simulink model "mapp_4_fir_4_str"  (R2018b)
settings: Solver=ode45  StartTime=0.0  StopTime=200  RelTol=1e-3  EnableMultiTasking=on
undefined symbols (not defined in the file or in its folder): CMD_ci_Re_0, CMD_ci_Re_21, CMD_ci_str_0, CMD_ci_str_1, CMD_ci_str_10, CMD_ci_str_11, CMD_ci_str_12, CMD_ci_str_13, CMD_ci_str_14, CMD_ci_str_15, CMD_ci_str_16, CMD_ci_str_17, CMD_ci_str_18, CMD_ci_str_19, CMD_ci_str_2, CMD_ci_str_20, CMD_ci_str_21, CMD_ci_str_3, CMD_ci_str_4, CMD_ci_str_5, CMD_ci_str_6, CMD_ci_str_7, CMD_ci_str_8, CMD_ci_str_9, CMD_decr_0, CMD_deka_down, CMD_deka_up, CMD_fb, CMD_FB_mult, CMD_Firprg_0, CMD_Firprg_1, CMD_gain, CMD_ind_mult, CMD_ind_mult_1, CMD_ind_mult_2, CMD_ind_mult_3, CMD_ind_mult_4, CMD_ind_stuk, CMD_ind_vol, CMD_ind_vol_1, CMD_ind_vol_2, CMD_ind_vol_3, CMD_ind_vol_4, CMD_init_dac, CMD_init_sw, CMD_molot_string, CMD_nl, CMD_nl_sl, CMD_omega_0, CMD_out_vol, CMD_param_0, CMD_param_5, CMD_pedal, CMD_reset, CMD_rst, CMD_shape_0, CMD_step_down, CMD_step_up, CMD_str_svertk, ind_mult_0 ... (+10)
libraries: xbsIndex_r4 x3300
(part 4 of 16)

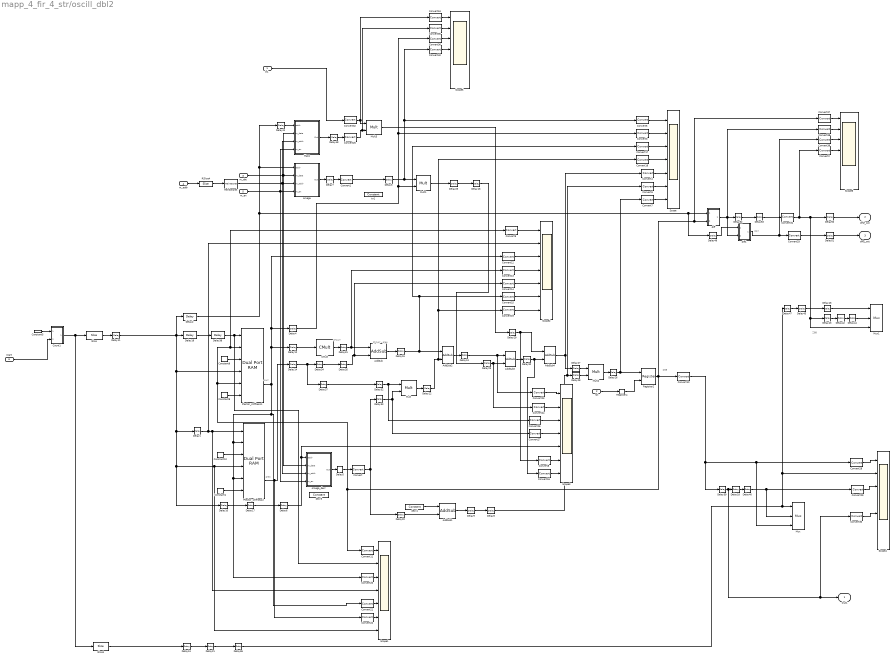
== system mapp_4_fir_4_str/oscill_dbl2 ==
  note: 2*curr - prev
  note: prev
  note: curr
  note: 2*curr
  note: Z59
  note: Z17
  note: Z88
  In1 : Inport
  rst : Inport  Port=2
  m_dat : Inport  Port=3
  m_addr : Inport  Port=4
  m_en : Inport  Port=5
  start : Inport  Port=6
  AddSub : xbsIndex_r4/AddSub  mode=Subtraction  use_carryin=off  use_carryout=off  en=off  latency=11  precision=Full  arith_type=Unsigned  n_bits=16  bin_pt=14  quantization=Truncate  overflow=Wrap  use_behavioral_HDL=off  hw_selection=DSP48  pipelined=on  dbl_ovrd=off  block_type=addsub
  AddSub1 : xbsIndex_r4/AddSub  mode=Subtraction  use_carryin=off  use_carryout=off  en=off  latency=11  precision=Full  arith_type=Unsigned  n_bits=25  bin_pt=0  quantization=Truncate  overflow=Wrap  use_behavioral_HDL=off  hw_selection=Fabric  pipelined=off  dbl_ovrd=off  block_type=addsub
  AddSub2 : xbsIndex_r4/AddSub  mode=Addition  use_carryin=off  use_carryout=off  en=off  latency=11  precision=Full  arith_type=Unsigned  n_bits=16  bin_pt=14  quantization=Truncate  overflow=Wrap  use_behavioral_HDL=off  hw_selection=Fabric  pipelined=off  dbl_ovrd=off  block_type=addsub
  AddSub3 : xbsIndex_r4/AddSub  mode=Subtraction  use_carryin=off  use_carryout=off  en=off  latency=11  precision=Full  arith_type=Unsigned  n_bits=16  bin_pt=14  quantization=Truncate  overflow=Wrap  use_behavioral_HDL=off  hw_selection=Fabric  pipelined=off  dbl_ovrd=off  block_type=addsub
  AddSub4 : xbsIndex_r4/AddSub  mode=Addition  use_carryin=off  use_carryout=off  en=off  latency=11  precision=Full  arith_type=Unsigned  n_bits=16  bin_pt=14  quantization=Truncate  overflow=Wrap  use_behavioral_HDL=off  hw_selection=Fabric  pipelined=off  dbl_ovrd=off  block_type=addsub
  CMult : xbsIndex_r4/CMult  const=2  gui_display_data_type=Floating-point  const_n_bits=16  const_bin_pt=14  float_type=Double  exp_bits=8  fraction_bits=24  en=off  latency=8  precision=Full  arith_type="Signed  (2's comp)"  n_bits=16  bin_pt=14  quantization=Truncate  overflow=Wrap  use_behavioral_HDL=off  mem_type=Distributed RAM  pipeline=on  dbl_ovrd=off  block_type=cmult
  Constant1 : xbsIndex_r4/Constant  const=0  gui_display_data_type=Boolean  arith_type=Boolean  n_bits=18  bin_pt=0  preci_type=Single  exp_width=8  frac_width=24  explicit_period=on  period=1  equ=P=C  opselect=C  inp2=PCIN>>17  opr=+  inp1=P  carry=CIN  dbl_ovrd=off  block_type=constant
      settings: block_version=VER_STRING_GOES_HERE
  Constant10 : xbsIndex_r4/Constant  const=1  gui_display_data_type=Boolean  arith_type=Boolean  n_bits=18  bin_pt=0  preci_type=Single  exp_width=8  frac_width=24  explicit_period=on  period=1  equ=P=C  opselect=C  inp2=PCIN>>17  opr=+  inp1=P  carry=CIN  dbl_ovrd=off  block_type=constant
      settings: block_version=VER_STRING_GOES_HERE
  Constant5 : xbsIndex_r4/Constant  const=169  gui_display_data_type=Fixed-point  arith_type=Unsigned  n_bits=12  bin_pt=0  preci_type=Single  exp_width=8  frac_width=24  explicit_period=off  period=1  equ=P=C  opselect=C  inp2=PCIN>>17  opr=+  inp1=P  carry=CIN  dbl_ovrd=off  block_type=constant
      settings: block_version=VER_STRING_GOES_HERE
  Constant8 : xbsIndex_r4/Constant  const=0  gui_display_data_type=Boolean  arith_type=Boolean  n_bits=18  bin_pt=0  preci_type=Single  exp_width=8  frac_width=24  explicit_period=on  period=1  equ=P=C  opselect=C  inp2=PCIN>>17  opr=+  inp1=P  carry=CIN  dbl_ovrd=off  block_type=constant
      settings: block_version=VER_STRING_GOES_HERE
  Constant9 : xbsIndex_r4/Constant  const=1  gui_display_data_type=Boolean  arith_type=Boolean  n_bits=18  bin_pt=0  preci_type=Single  exp_width=8  frac_width=24  explicit_period=on  period=1  equ=P=C  opselect=C  inp2=PCIN>>17  opr=+  inp1=P  carry=CIN  dbl_ovrd=off  block_type=constant
      settings: block_version=VER_STRING_GOES_HERE
  Convert{,1,25,32} (4 alike) : xbsIndex_r4/Convert  gui_display_data_type=Floating-point  arith_type=Floating-point  n_bits=16  bin_pt=14  float_type=Double  exp_bits=8  fraction_bits=24  quantization=Truncate  overflow=Wrap  en=off  latency=12  pipeline=off  dbl_ovrd=off  block_type=convert
  Convert10 : xbsIndex_r4/Convert  gui_display_data_type=Floating-point  arith_type=Floating-point  n_bits=16  bin_pt=14  float_type=Single  exp_bits=8  fraction_bits=24  quantization=Truncate  overflow=Wrap  en=off  latency=12  pipeline=off  dbl_ovrd=off  block_type=convert
  Convert{3..9,11..24,26..27,34..40} (30 alike) : xbsIndex_r4/Convert  gui_display_data_type=Floating-point  arith_type=Floating-point  n_bits=16  bin_pt=14  float_type=Double  exp_bits=8  fraction_bits=24  quantization=Truncate  overflow=Wrap  en=off  latency=0  pipeline=off  dbl_ovrd=off  block_type=convert
  Convert{2,28..30} (4 alike) : xbsIndex_r4/Convert  gui_display_data_type=Floating-point  arith_type=Floating-point  n_bits=16  bin_pt=14  float_type=Single  exp_bits=8  fraction_bits=24  quantization=Truncate  overflow=Wrap  en=off  latency=0  pipeline=off  dbl_ovrd=off  block_type=convert
  Convert31 : xbsIndex_r4/Convert  gui_display_data_type=Floating-point  arith_type=Floating-point  n_bits=16  bin_pt=14  float_type=Single  exp_bits=8  fraction_bits=24  quantization=Truncate  overflow=Wrap  en=off  latency=12  pipeline=off  dbl_ovrd=off  block_type=convert
  Convert33 : xbsIndex_r4/Convert  gui_display_data_type=Floating-point  arith_type=Floating-point  n_bits=16  bin_pt=14  float_type=Single  exp_bits=8  fraction_bits=24  quantization=Truncate  overflow=Wrap  en=off  latency=12  pipeline=off  dbl_ovrd=off  block_type=convert
  Count1 : Subsystem
  Delay{1,3,16,33} (4 alike) : xbsIndex_r4/Delay  rst=off  infoeditControl=Selection of Reset will increase slice count due to use of real FFs and instead of SRLs  en=off  latency=2  reg_retiming=on  dbl_ovrd=off  block_type=delay
      settings: xl_area=[16 32 0 0 0 0 0]  block_version=VER_STRING_GOES_HERE
  Delay{2,5..7,9..10,12..15,22..32,35..36,38..40,43..44,46..48,50..51,53} (34 alike) : xbsIndex_r4/Delay  rst=off  infoeditControl=Selection of Reset will increase slice count due to use of real FFs and instead of SRLs  en=off  latency=1  reg_retiming=on  dbl_ovrd=off  block_type=delay
      Delay10 settings: xl_area=[16 32 0 0 0 0 0]  block_version=VER_STRING_GOES_HERE
      Delay12 settings: xl_area=[16 32 0 0 0 0 0]  block_version=VER_STRING_GOES_HERE
      Delay13 settings: xl_area=[16 32 0 0 0 0 0]  block_version=VER_STRING_GOES_HERE
      Delay14 settings: xl_area=[16 32 0 0 0 0 0]  block_version=VER_STRING_GOES_HERE
      Delay15 settings: xl_area=[16 32 0 0 0 0 0]  block_version=VER_STRING_GOES_HERE
      Delay2 settings: xl_area=[1 1 0 0 0 0 0]  block_version=8.2-EVAL
      Delay22 settings: xl_area=[16 32 0 0 0 0 0]  block_version=VER_STRING_GOES_HERE
      Delay23 settings: xl_area=[16 32 0 0 0 0 0]  block_version=VER_STRING_GOES_HERE
      Delay24 settings: xl_area=[16 32 0 0 0 0 0]  block_version=VER_STRING_GOES_HERE
      Delay25 settings: xl_area=[16 32 0 0 0 0 0]  block_version=VER_STRING_GOES_HERE
      Delay26 settings: xl_area=[16 32 0 0 0 0 0]  block_version=VER_STRING_GOES_HERE
      Delay27 settings: xl_area=[16 32 0 0 0 0 0]  block_version=VER_STRING_GOES_HERE
      Delay28 settings: xl_area=[16 32 0 0 0 0 0]  block_version=VER_STRING_GOES_HERE
      Delay29 settings: xl_area=[16 32 0 0 0 0 0]  block_version=VER_STRING_GOES_HERE
      Delay30 settings: xl_area=[16 32 0 0 0 0 0]  block_version=VER_STRING_GOES_HERE
      Delay31 settings: xl_area=[16 32 0 0 0 0 0]  block_version=VER_STRING_GOES_HERE
      Delay32 settings: xl_area=[16 32 0 0 0 0 0]  block_version=VER_STRING_GOES_HERE
      Delay35 settings: xl_area=[16 32 0 0 0 0 0]  block_version=VER_STRING_GOES_HERE
      Delay36 settings: xl_area=[16 32 0 0 0 0 0]  block_version=VER_STRING_GOES_HERE
      Delay38 settings: xl_area=[1 1 0 0 0 0 0]  block_version=8.2-EVAL
      Delay39 settings: xl_area=[16 32 0 0 0 0 0]  block_version=VER_STRING_GOES_HERE
      Delay40 settings: xl_area=[16 32 0 0 0 0 0]  block_version=VER_STRING_GOES_HERE
      Delay43 settings: xl_area=[16 32 0 0 0 0 0]  block_version=VER_STRING_GOES_HERE
      Delay44 settings: xl_area=[16 32 0 0 0 0 0]  block_version=VER_STRING_GOES_HERE
      Delay46 settings: xl_area=[16 32 0 0 0 0 0]  block_version=VER_STRING_GOES_HERE
      Delay47 settings: xl_area=[16 32 0 0 0 0 0]  block_version=VER_STRING_GOES_HERE
      Delay48 settings: xl_area=[16 32 0 0 0 0 0]  block_version=VER_STRING_GOES_HERE
      Delay5 settings: xl_area=[16 32 0 0 0 0 0]  block_version=VER_STRING_GOES_HERE
      Delay50 settings: xl_area=[16 32 0 0 0 0 0]  block_version=VER_STRING_GOES_HERE
      Delay51 settings: xl_area=[16 32 0 0 0 0 0]  block_version=VER_STRING_GOES_HERE
      Delay53 settings: xl_area=[16 32 0 0 0 0 0]  block_version=VER_STRING_GOES_HERE
      Delay6 settings: xl_area=[16 32 0 0 0 0 0]  block_version=VER_STRING_GOES_HERE
      Delay7 settings: xl_area=[16 32 0 0 0 0 0]  block_version=VER_STRING_GOES_HERE
      Delay9 settings: xl_area=[16 32 0 0 0 0 0]  block_version=VER_STRING_GOES_HERE
  Delay11 : xbsIndex_r4/Delay  rst=off  infoeditControl=Selection of Reset will increase slice count due to use of real FFs and instead of SRLs  en=off  latency=16  reg_retiming=on  dbl_ovrd=off  block_type=delay
      settings: xl_area=[16 32 0 0 0 0 0]  block_version=VER_STRING_GOES_HERE
  Delay17 : xbsIndex_r4/Delay  rst=off  infoeditControl=Selection of Reset will increase slice count due to use of real FFs and instead of SRLs  en=off  latency=246  reg_retiming=on  dbl_ovrd=off  block_type=delay
      settings: xl_area=[16 32 0 0 0 0 0]  block_version=VER_STRING_GOES_HERE
  Delay18 : xbsIndex_r4/Delay  rst=off  infoeditControl=Selection of Reset will increase slice count due to use of real FFs and instead of SRLs  en=off  latency=254  reg_retiming=on  dbl_ovrd=off  block_type=delay
      settings: xl_area=[16 32 0 0 0 0 0]  block_version=VER_STRING_GOES_HERE
  Delay19 : xbsIndex_r4/Delay  rst=off  infoeditControl=Selection of Reset will increase slice count due to use of real FFs and instead of SRLs  en=off  latency=77  reg_retiming=on  dbl_ovrd=off  block_type=delay
      settings: xl_area=[1 1 0 0 0 0 0]  block_version=8.2-EVAL
  Delay20 : xbsIndex_r4/Delay  rst=off  infoeditControl=Selection of Reset will increase slice count due to use of real FFs and instead of SRLs  en=off  latency=12  reg_retiming=on  dbl_ovrd=off  block_type=delay
      settings: xl_area=[16 32 0 0 0 0 0]  block_version=VER_STRING_GOES_HERE
  Delay21 : xbsIndex_r4/Delay  rst=off  infoeditControl=Selection of Reset will increase slice count due to use of real FFs and instead of SRLs  en=off  latency=41 + 64  reg_retiming=on  dbl_ovrd=off  block_type=delay
      settings: xl_area=[16 32 0 0 0 0 0]  block_version=VER_STRING_GOES_HERE
  Delay34 : xbsIndex_r4/Delay  rst=off  infoeditControl=Selection of Reset will increase slice count due to use of real FFs and instead of SRLs  en=off  latency=8  reg_retiming=on  dbl_ovrd=off  block_type=delay
      settings: xl_area=[16 32 0 0 0 0 0]  block_version=VER_STRING_GOES_HERE
  Delay37 : xbsIndex_r4/Delay  rst=off  infoeditControl=Selection of Reset will increase slice count due to use of real FFs and instead of SRLs  en=off  latency=3  reg_retiming=on  dbl_ovrd=off  block_type=delay
      settings: xl_area=[16 32 0 0 0 0 0]  block_version=VER_STRING_GOES_HERE
  Delay4 : xbsIndex_r4/Delay  rst=off  infoeditControl=Selection of Reset will increase slice count due to use of real FFs and instead of SRLs  en=off  latency=14  reg_retiming=on  dbl_ovrd=off  block_type=delay
      settings: xl_area=[16 32 0 0 0 0 0]  block_version=VER_STRING_GOES_HERE
  Delay41 : xbsIndex_r4/Delay  rst=off  infoeditControl=Selection of Reset will increase slice count due to use of real FFs and instead of SRLs  en=off  latency=17  reg_retiming=on  dbl_ovrd=off  block_type=delay
      settings: xl_area=[16 32 0 0 0 0 0]  block_version=VER_STRING_GOES_HERE
  Delay42 : xbsIndex_r4/Delay  rst=off  infoeditControl=Selection of Reset will increase slice count due to use of real FFs and instead of SRLs  en=off  latency=126  reg_retiming=on  dbl_ovrd=off  block_type=delay
      settings: xl_area=[16 32 0 0 0 0 0]  block_version=VER_STRING_GOES_HERE
  Delay45 : xbsIndex_r4/Delay  rst=off  infoeditControl=Selection of Reset will increase slice count due to use of real FFs and instead of SRLs  en=off  latency=15  reg_retiming=on  dbl_ovrd=off  block_type=delay
      settings: xl_area=[16 32 0 0 0 0 0]  block_version=VER_STRING_GOES_HERE
  Delay49 : xbsIndex_r4/Delay  rst=off  infoeditControl=Selection of Reset will increase slice count due to use of real FFs and instead of SRLs  en=off  latency=17  reg_retiming=on  dbl_ovrd=off  block_type=delay
      settings: xl_area=[16 32 0 0 0 0 0]  block_version=VER_STRING_GOES_HERE
  Delay52 : xbsIndex_r4/Delay  rst=off  infoeditControl=Selection of Reset will increase slice count due to use of real FFs and instead of SRLs  en=off  latency=16  reg_retiming=on  dbl_ovrd=off  block_type=delay
      settings: xl_area=[16 32 0 0 0 0 0]  block_version=VER_STRING_GOES_HERE
  Delay8 : xbsIndex_r4/Delay  rst=off  infoeditControl=Selection of Reset will increase slice count due to use of real FFs and instead of SRLs  en=off  latency=30  reg_retiming=on  dbl_ovrd=off  block_type=delay
      settings: xl_area=[16 32 0 0 0 0 0]  block_version=VER_STRING_GOES_HERE
  Mass : Subsystem
  Mult : xbsIndex_r4/Mult  precision=Full  arith_type="Signed  (2's comp)"  n_bits=48  bin_pt=48  quantization=Truncate  overflow=Wrap  en=off  latency=16  use_behavioral_HDL=off  opt=Speed  use_embedded=on  optimum_pipeline=on  pipeline=on  dbl_ovrd=off  use_rpm=on  placement_style=Triangular  block_type=mult
      settings: block_version=9.1.01-EVAL
  Mult1 : xbsIndex_r4/Mult  precision=Full  arith_type="Signed  (2's comp)"  n_bits=48  bin_pt=48  quantization=Truncate  overflow=Wrap  en=off  latency=16  use_behavioral_HDL=on  opt=Speed  use_embedded=on  optimum_pipeline=on  pipeline=on  dbl_ovrd=off  use_rpm=on  placement_style=Triangular  block_type=mult
      settings: block_version=9.1.01-EVAL
  Mult2 : xbsIndex_r4/Mult  precision=Full  arith_type="Signed  (2's comp)"  n_bits=48  bin_pt=48  quantization=Truncate  overflow=Wrap  en=off  latency=16  use_behavioral_HDL=on  opt=Speed  use_embedded=on  optimum_pipeline=on  pipeline=on  dbl_ovrd=off  use_rpm=on  placement_style=Triangular  block_type=mult
      settings: block_version=9.1.01-EVAL
  Mult3 : xbsIndex_r4/Mult  precision=Full  arith_type="Signed  (2's comp)"  n_bits=48  bin_pt=48  quantization=Truncate  overflow=Wrap  en=off  latency=16  use_behavioral_HDL=on  opt=Speed  use_embedded=on  optimum_pipeline=on  pipeline=on  dbl_ovrd=off  use_rpm=on  placement_style=Triangular  block_type=mult
      settings: block_version=9.1.01-EVAL
  Mux : xbsIndex_r4/Mux  inputs=2  en=off  latency=0  precision=Full  arith_type=Unsigned  n_bits=16  bin_pt=14  quantization=Truncate  overflow=Wrap  dbl_ovrd=off  block_type=mux
  Mux1 : xbsIndex_r4/Mux  inputs=2  en=off  latency=0  precision=Full  arith_type=Unsigned  n_bits=16  bin_pt=14  quantization=Truncate  overflow=Wrap  dbl_ovrd=off  block_type=mux
  Plector_stiffness1 : xbsIndex_r4/Dual Port RAM  depth=256  initVector=zeros  distributed_mem=Block RAM  init_a=0  init_b=0  rst_a=off  rst_b=off  en_a=off  en_b=off  latency=2  write_mode_A=Read Before Write  write_mode_B=Read Before Write  optimize=Area  dbl_ovrd=off  block_type=dpram
      settings: block_version=10.1.1
  Plector_stiffness2 : xbsIndex_r4/Dual Port RAM  depth=256  initVector=zeros  distributed_mem=Block RAM  init_a=0  init_b=0  rst_a=off  rst_b=off  en_a=off  en_b=off  latency=2  write_mode_A=Read Before Write  write_mode_B=Read Before Write  optimize=Area  dbl_ovrd=off  block_type=dpram
      settings: block_version=10.1.1
  RSlice4 : xbsIndex_r4/Slice  nbits=8  boolean_output=off  mode=Lower Bit Location + Width  bit1=0  base1=MSB of Input  bit0=0  base0=LSB of Input  dbl_ovrd=off  block_type=slice
      settings: block_version=VER_STRING_GOES_HERE
  Register2 : xbsIndex_r4/Register  init=0  rst=on  en=off  dbl_ovrd=off  block_type=register
  Register4 : xbsIndex_r4/Register  init=0  rst=off  en=off  dbl_ovrd=off  block_type=register
  Reinterpret : xbsIndex_r4/Reinterpret  force_arith_type=off  arith_type=Unsigned  force_bin_pt=off  bin_pt=0  block_type=reinterpret
  Scope{,1..6} (7 alike) : Scope  NumInputPorts=7
  Slice : xbsIndex_r4/Slice  nbits=8  boolean_output=off  mode=Lower Bit Location + Width  bit1=0  base1=MSB of Input  bit0=0  base0=LSB of Input  dbl_ovrd=off  block_type=slice
  Slice1 : xbsIndex_r4/Slice  nbits=1  boolean_output=off  mode=Lower Bit Location + Width  bit1=0  base1=MSB of Input  bit0=7  base0=LSB of Input  dbl_ovrd=off  block_type=slice
  decr3 : xbsIndex_r4/Constant  const=0.01  gui_display_data_type=Floating-point  arith_type=Floating-point  n_bits=25  bin_pt=0  preci_type=Double  exp_width=8  frac_width=24  explicit_period=on  period=1  equ=P=C  opselect=C  inp2=PCIN>>17  opr=+  inp1=P  carry=CIN  dbl_ovrd=off  block_type=constant
      settings: block_version=VER_STRING_GOES_HERE
  decr4 : xbsIndex_r4/Constant  const=1  gui_display_data_type=Floating-point  arith_type=Floating-point  n_bits=25  bin_pt=0  preci_type=Double  exp_width=8  frac_width=24  explicit_period=on  period=1  equ=P=C  opselect=C  inp2=PCIN>>17  opr=+  inp1=P  carry=CIN  dbl_ovrd=off  block_type=constant
      settings: block_version=VER_STRING_GOES_HERE
  diff : Subsystem
  diff1 : Subsystem
  omega : Subsystem
  omega_decr : Subsystem
  tn1 : xbsIndex_r4/Constant  const=1  gui_display_data_type=Floating-point  arith_type=Floating-point  n_bits=18  bin_pt=0  preci_type=Double  exp_width=8  frac_width=24  explicit_period=on  period=1  equ=P=C  opselect=C  inp2=PCIN>>17  opr=+  inp1=P  carry=CIN  dbl_ovrd=off  block_type=constant
      settings: block_version=VER_STRING_GOES_HERE
  Out1 : Outport
  dif1f_out : Outport  Port=2
  diff2_out : Outport  Port=3
  wires:
  Convert40/1 -> Scope5/4
  Convert36/1 -> Scope5/3
  Convert34/1 -> Scope5/1
  Convert35/1 -> Scope5/2
  Convert39/1 -> Scope6/3
  Convert38/1 -> Scope6/2
  Convert37/1 -> Scope6/1
  Delay49/1 -> diff1/1(In1)
  Convert25/1 -> Mult3/2, Convert35/1
  Convert32/1 -> Convert34/1, Mult3/1
  Mass/1(Out) -> Delay48/1
  Delay48/1 -> Convert25/1
  Delay41/1 -> Mass/1(addr)
  Delay36/1 -> Scope4/2, Delay47/1, Mux/1
  Delay42/1 -> Delay44/1
  Delay43/1 -> Delay42/1
  Delay44/1 -> Mux1/2
  diff/1(first_derr) -> Convert38/1, Delay52/1, diff1/2(In2)
  Delay45/1 -> Delay46/1
  Delay46/1 -> Mux1/1
  Delay47/1 -> Delay45/1
  Delay39/1 -> Convert30/1, Out1/1, Delay18/1
  Convert30/1 -> Scope4/5
  Delay40/1 -> Convert29/1, Mux/2
  Delay24/1 -> Delay21/1
  Delay21/1 -> Delay36/1
  Convert29/1 -> Scope4/3
  Delay18/1 -> Delay40/1
  Slice1/1 -> Delay24/1
  Convert28/1 -> Scope4/1
  Delay10/1 -> Delay17/1
  Delay20/1 -> AddSub1/2
  Delay17/1 -> Delay6/1
  Convert27/1 -> Scope3/4
  Convert26/1 -> Scope3/3
  Convert18/1 -> Scope/4
  Convert17/1 -> Scope/3
  Delay1/1 -> Plector_stiffness2/1, Scope1/4, Scope2/2
  Convert5/1 -> Scope/1
  Convert4/1 -> Scope/5
  Delay2/1 -> omega/1(addr), Delay41/1, diff/1(In1), Delay49/1
  Delay38/1 -> Plector_stiffness1/1, Scope1/2
  Convert3/1 -> Scope/2
  Convert24/1 -> Scope3/2
  Convert23/1 -> Scope3/1
  Delay37/1 -> Delay32/1
  Convert22/1 -> Scope1/6
  Convert21/1 -> Scope1/5
  Plector_stiffness1/2 -> Convert21/1, Plector_stiffness2/2, Plector_stiffness2/5, Convert20/1, Delay4/1, Convert12/1, Delay12/1
  Convert20/1 -> Scope1/3
  Convert19/1 -> Scope2/7
  Convert7/1 -> Scope/7
  Convert6/1 -> Scope/6
  Constant5/1 -> Count1/1(In1)
  Convert1/1 -> Delay3/1
  Delay4/1 -> Mult1/2, Convert3/1, Convert36/1
  Convert15/1 -> Scope2/6
  Convert14/1 -> Scope2/5
  Convert13/1 -> Scope2/4
  Convert12/1 -> Scope2/3
  Convert9/1 -> Scope2/1
  In1/1 -> Convert32/1
  Delay35/1 -> AddSub/2, Convert14/1
  Delay34/1 -> Delay35/1
  Delay33/1 -> Mult/2, Convert27/1
  Delay32/1 -> Convert26/1, Mult/1
  Delay31/1 -> AddSub/1, Convert13/1
  Delay30/1 -> Convert16/1, AddSub4/2
  Delay29/1 -> Convert8/1, AddSub4/1
  Delay28/1 -> Mult2/2
  Delay27/1 -> Mult2/1
  Delay26/1 -> Register2/1, Convert7/1
  Delay25/1 -> Delay16/1
  Delay7/1 -> Convert1/1
  Delay5/1 -> Convert/1
  Delay23/1 -> AddSub3/2, Convert24/1
  Convert11/1 -> Scope1/1
  decr4/1 -> AddSub1/1
  Delay11/1 -> Delay19/1, Delay2/1, Plector_stiffness1/4, Plector_stiffness2/4, Scope1/7, Delay10/1, Delay1/1
  Register4/1 -> Register2/2
  rst/1 -> Register4/1
  Delay6/1 -> omega_decr/1(addr), Scope3/5
  CMult/1 -> Delay31/1
  Delay12/1 -> CMult/1
  Delay19/1 -> Delay38/1
  Constant9/1 -> Plector_stiffness1/3
  Count1/1(Out1) -> Slice/1, Slice1/1
  omega/1(Out) -> Delay7/1
  Plector_stiffness2/2 -> Delay14/1, Convert22/1
  AddSub1/1 -> Delay9/1
  Convert/1 -> Delay33/1, Delay20/1
  Register2/1 -> Convert10/1, Plector_stiffness1/2, Convert9/1, Plector_stiffness1/5, Convert11/1, Convert37/1, diff/2(In2)
  Delay8/1 -> Delay28/1, Convert6/1
  Constant8/1 -> Plector_stiffness1/6
  Constant1/1 -> Plector_stiffness2/6
  AddSub/1 -> Delay15/1
  AddSub2/1 -> Delay13/1
  Slice/1 -> Delay11/1
  AddSub4/1 -> Delay27/1, Convert4/1
  Constant10/1 -> Plector_stiffness2/3
  Delay9/1 -> Delay8/1
  omega_decr/1(Out) -> Delay5/1
  Delay14/1 -> Delay34/1, Delay37/1
  Delay13/1 -> AddSub3/1, Convert23/1
  Delay3/1 -> Mult1/1, Convert5/1, Convert40/1
  Delay16/1 -> Delay23/1
  Mult1/1 -> Delay25/1
  m_dat/1 -> omega/2(m_data), omega_decr/2(m_data), Mass/2(m_data)
  m_en/1 -> omega/4(m_en), omega_decr/4(m_en), Mass/4(m_en)
  m_addr/1 -> RSlice4/1
  RSlice4/1 -> Reinterpret/1
  Reinterpret/1 -> omega/3(m_addr), Mass/3(m_addr), omega_decr/3(m_addr)
  Mult3/1 -> Delay29/1
  Delay15/1 -> Convert15/1, Convert17/1, AddSub2/1
  Mult/1 -> Delay22/1
  Mult2/1 -> Delay26/1
  AddSub3/1 -> Delay30/1
  Convert10/1 -> Convert28/1, Mux/3, Delay39/1
  Delay22/1 -> AddSub2/2, Convert19/1, Convert18/1
  Convert8/1 -> Scope3/6
  Convert16/1 -> Scope3/7
  start/1 -> Count1/2(start)
  diff1/1(first_derr) -> Convert33/1, Convert39/1
  Convert2/1 -> Scope6/4
  Delay50/1 -> dif1f_out/1
  Delay51/1 -> diff2_out/1
  Delay52/1 -> Delay53/1
  Convert31/1 -> Convert2/1, Delay43/1, Mux1/3, Delay50/1
  Delay53/1 -> Convert31/1
  Convert33/1 -> Delay51/1

== system mapp_4_fir_4_str/MUX0/Count2 ==
  In1 : Inport
  start : Inport  Port=2
  Constant1 : xbsIndex_r4/Constant  const=1  gui_display_data_type=Fixed-point  arith_type=Boolean  n_bits=5  bin_pt=0  preci_type=Single  exp_width=8  frac_width=24  explicit_period=off  period=1  equ=P=C  opselect=C  inp2=PCIN>>17  opr=+  inp1=P  carry=CIN  dbl_ovrd=off  block_type=constant
      settings: block_version=VER_STRING_GOES_HERE
  Counter1 : xbsIndex_r4/Counter  cnt_type=Free Running  cnt_to=1  operation=Up  start_count=0  cnt_by_val=1  arith_type=Unsigned  n_bits=11  bin_pt=0  load_pin=off  rst=off  en=on  explicit_period=on  period=1  use_behavioral_HDL=off  implementation=Fabric  use_rpm=off  dbl_ovrd=off  block_type=counter
      settings: block_version=8.2.02
  Counter2 : xbsIndex_r4/Counter  cnt_type=Free Running  cnt_to=num_point_256*num_str0*1 - 1  operation=Up  start_count=0  cnt_by_val=1  arith_type=Unsigned  n_bits=10  bin_pt=0  load_pin=off  rst=off  en=on  explicit_period=on  period=1  use_behavioral_HDL=off  implementation=Fabric  use_rpm=off  dbl_ovrd=off  block_type=counter
      settings: block_version=8.2.02
  Delay2 : xbsIndex_r4/Delay  rst=off  infoeditControl=Selection of Reset will increase slice count due to use of real FFs and instead of SRLs  en=off  latency=1  reg_retiming=on  dbl_ovrd=off  block_type=delay
      settings: xl_area=[2 4 0 4 0 0 0]  block_version=8.2-EVAL
  RSlice1 : xbsIndex_r4/Slice  nbits=ceil(log2(2*num_str0))  boolean_output=off  mode=Lower Bit Location + Width  bit1=0  base1=MSB of Input  bit0=6  base0=LSB of Input  dbl_ovrd=off  block_type=slice
      settings: block_version=VER_STRING_GOES_HERE
  RSlice2 : xbsIndex_r4/Slice  nbits=2  boolean_output=off  mode=Upper Bit Location + Width  bit1=0  base1=MSB of Input  bit0=7  base0=LSB of Input  dbl_ovrd=off  block_type=slice
      settings: block_version=VER_STRING_GOES_HERE
  Register6 : xbsIndex_r4/Register  init=0  rst=off  en=on  dbl_ovrd=off  block_type=register
  Relational1 : xbsIndex_r4/Relational  mode=a=b  op_type=Bool  en=off  latency=1  dbl_ovrd=off  block_type=relational
      settings: xl_area=[4 1 0 7 0 0 0]  block_version=VER_STRING_GOES_HERE
  Scope1 : Scope  NumInputPorts=8
  Out1 : Outport
  Out2 : Outport  Port=2
  Out3 : Outport  Port=3
  wires:
  start/1 -> Delay2/1
  Delay2/1 -> Counter1/1
  Counter2/1 -> RSlice2/1, RSlice1/1, Out1/1
  Counter1/1 -> Relational1/1
  Constant1/1 -> Register6/1
  Relational1/1 -> Register6/2
  Register6/1 -> Counter2/1
  In1/1 -> Relational1/2
  RSlice1/1 -> Out2/1
  RSlice2/1 -> Out3/1

== system mapp_4_fir_4_str/MUX0/add_0 ==
  note: Isin
  Re : Inport
  rst : Inport  Port=2
  start : Inport  Port=3
  AddSub : xbsIndex_r4/AddSub  mode=Addition  use_carryin=off  use_carryout=off  en=off  latency=11  precision=Full  arith_type=Unsigned  n_bits=16  bin_pt=14  quantization=Truncate  overflow=Wrap  use_behavioral_HDL=off  hw_selection=Fabric  pipelined=off  dbl_ovrd=off  block_type=addsub
  Constant1 : xbsIndex_r4/Constant  const=2  gui_display_data_type=Fixed-point  arith_type=Unsigned  n_bits=2  bin_pt=0  preci_type=Single  exp_width=8  frac_width=24  explicit_period=on  period=1  equ=P=C  opselect=C  inp2=PCIN>>17  opr=+  inp1=P  carry=CIN  dbl_ovrd=off  block_type=constant
      settings: block_version=VER_STRING_GOES_HERE
  Constant11 : xbsIndex_r4/Constant  const=382  gui_display_data_type=Fixed-point  arith_type=Unsigned  n_bits=12  bin_pt=0  preci_type=Single  exp_width=8  frac_width=24  explicit_period=off  period=1  equ=P=C  opselect=C  inp2=PCIN>>17  opr=+  inp1=P  carry=CIN  dbl_ovrd=off  block_type=constant
      settings: block_version=VER_STRING_GOES_HERE
  Constant15 : xbsIndex_r4/Constant  const=0  gui_display_data_type=Floating-point  arith_type=Floating-point  n_bits=48  bin_pt=0  preci_type=Single  exp_width=8  frac_width=24  explicit_period=on  period=1  equ=P=C  opselect=C  inp2=PCIN>>17  opr=+  inp1=P  carry=CIN  dbl_ovrd=off  block_type=constant
      settings: block_version=VER_STRING_GOES_HERE
  Constant2 : xbsIndex_r4/Constant  const=0  gui_display_data_type=Fixed-point  arith_type=Boolean  n_bits=16  bin_pt=14  preci_type=Single  exp_width=8  frac_width=24  explicit_period=on  period=1  equ=P=C  opselect=C  inp2=PCIN>>17  opr=+  inp1=P  carry=CIN  dbl_ovrd=off  block_type=constant
      settings: block_version=VER_STRING_GOES_HERE
  Constant3 : xbsIndex_r4/Constant  const=1  gui_display_data_type=Boolean  arith_type=Boolean  n_bits=5  bin_pt=0  preci_type=Single  exp_width=8  frac_width=24  explicit_period=off  period=1  equ=P=C  opselect=C  inp2=PCIN>>17  opr=+  inp1=P  carry=CIN  dbl_ovrd=off  block_type=constant
      settings: block_version=VER_STRING_GOES_HERE
  Constant4 : xbsIndex_r4/Constant  const=1  gui_display_data_type=Fixed-point  arith_type=Unsigned  n_bits=1  bin_pt=0  preci_type=Single  exp_width=8  frac_width=24  explicit_period=off  period=1  equ=P=C  opselect=C  inp2=PCIN>>17  opr=+  inp1=P  carry=CIN  dbl_ovrd=off  block_type=constant
      settings: block_version=VER_STRING_GOES_HERE
  Constant6 : xbsIndex_r4/Constant  const=3  gui_display_data_type=Fixed-point  arith_type=Unsigned  n_bits=2  bin_pt=0  preci_type=Single  exp_width=8  frac_width=24  explicit_period=on  period=1  equ=P=C  opselect=C  inp2=PCIN>>17  opr=+  inp1=P  carry=CIN  dbl_ovrd=off  block_type=constant
      settings: block_version=VER_STRING_GOES_HERE
  Constant8 : xbsIndex_r4/Constant  const=1  gui_display_data_type=Fixed-point  arith_type=Boolean  n_bits=16  bin_pt=14  preci_type=Single  exp_width=8  frac_width=24  explicit_period=on  period=1  equ=P=C  opselect=C  inp2=PCIN>>17  opr=+  inp1=P  carry=CIN  dbl_ovrd=off  block_type=constant
      settings: block_version=VER_STRING_GOES_HERE
  Convert1 : xbsIndex_r4/Convert  gui_display_data_type=Fixed-point  arith_type=Boolean  n_bits=48  bin_pt=48  float_type=Single  exp_bits=8  fraction_bits=24  quantization=Truncate  overflow=Saturate  en=off  latency=0  pipeline=off  dbl_ovrd=off  block_type=convert
      settings: xl_area=[0 0 0 0 0 0 0]  block_version=8.2-EVAL
  Convert{2..8} (7 alike) : xbsIndex_r4/Convert  gui_display_data_type=Floating-point  arith_type=Floating-point  n_bits=16  bin_pt=14  float_type=Single  exp_bits=8  fraction_bits=24  quantization=Truncate  overflow=Wrap  en=off  latency=0  pipeline=off  dbl_ovrd=off  block_type=convert
  Isin : xbsIndex_r4/Dual Port RAM  depth=num_harm_32  initVector=zeros  distributed_mem=Block RAM  init_a=0  init_b=0  rst_a=off  rst_b=off  en_a=off  en_b=off  latency=1  write_mode_A=Read Before Write  write_mode_B=Read Before Write  optimize=Speed  dbl_ovrd=off  block_type=dpram
      settings: xl_area=[96 48 48 144 0 0 0]  block_version=VER_STRING_GOES_HERE
  Mux : xbsIndex_r4/Mux  inputs=2  en=off  latency=0  precision=Full  arith_type=Unsigned  n_bits=16  bin_pt=14  quantization=Truncate  overflow=Wrap  dbl_ovrd=off  block_type=mux
  Register1 : xbsIndex_r4/Register  init=0  rst=on  en=off  dbl_ovrd=off  block_type=register
      settings: xl_area=[18 36 0 0 0 0 0]  block_version=VER_STRING_GOES_HERE
  Register{2,9..13,17} (7 alike) : xbsIndex_r4/Register  init=0  rst=off  en=off  dbl_ovrd=off  block_type=register
  Register6 : xbsIndex_r4/Register  init=0  rst=off  en=on  dbl_ovrd=off  block_type=register
  Relational : xbsIndex_r4/Relational  mode=a=b  op_type=Bool  en=off  latency=0  dbl_ovrd=off  block_type=relational
  Relational1 : xbsIndex_r4/Relational  mode=a=b  op_type=Bool  en=off  latency=0  dbl_ovrd=off  block_type=relational
  Relational2 : xbsIndex_r4/Relational  mode=a=b  op_type=Bool  en=off  latency=1  dbl_ovrd=off  block_type=relational
      settings: xl_area=[4 1 0 7 0 0 0]  block_version=VER_STRING_GOES_HERE
  Scope1 : Scope  NumInputPorts=6
  Scope2 : Scope  NumInputPorts=7
  Scope3 : Scope  NumInputPorts=6
  Single Port RAM : xbsIndex_r4/Single Port RAM  depth=num_harm_32  initVector=zeros  distributed_mem=Block RAM  write_mode=Read After Write  rst=off  init_reg=0  en=off  latency=1  optimize=Area  dbl_ovrd=off  block_type=spram
  Subsystem3 : Subsystem
  curr1 : xbsIndex_r4/Delay  rst=off  infoeditControl=Selection of Reset will increase slice count due to use of real FFs and instead of SRLs  en=off  latency=5  reg_retiming=on  dbl_ovrd=off  block_type=delay
      settings: xl_area=[17 33 0 33 0 0 0]  block_version=VER_STRING_GOES_HERE
  curr11 : xbsIndex_r4/Delay  rst=off  infoeditControl=Selection of Reset will increase slice count due to use of real FFs and instead of SRLs  en=off  latency=1  reg_retiming=on  dbl_ovrd=off  block_type=delay
      settings: xl_area=[17 33 0 33 0 0 0]  block_version=VER_STRING_GOES_HERE
  curr12 : xbsIndex_r4/Delay  rst=off  infoeditControl=Selection of Reset will increase slice count due to use of real FFs and instead of SRLs  en=off  latency=1  reg_retiming=on  dbl_ovrd=off  block_type=delay
      settings: xl_area=[17 33 0 33 0 0 0]  block_version=VER_STRING_GOES_HERE
  curr19 : xbsIndex_r4/Delay  rst=off  infoeditControl=Selection of Reset will increase slice count due to use of real FFs and instead of SRLs  en=off  latency=18  reg_retiming=on  dbl_ovrd=off  block_type=delay
      settings: xl_area=[17 33 0 33 0 0 0]  block_version=VER_STRING_GOES_HERE
  curr2 : xbsIndex_r4/Delay  rst=off  infoeditControl=Selection of Reset will increase slice count due to use of real FFs and instead of SRLs  en=off  latency=39  reg_retiming=on  dbl_ovrd=off  block_type=delay
      settings: xl_area=[17 33 0 33 0 0 0]  block_version=VER_STRING_GOES_HERE
  curr4 : xbsIndex_r4/Delay  rst=off  infoeditControl=Selection of Reset will increase slice count due to use of real FFs and instead of SRLs  en=off  latency=21  reg_retiming=on  dbl_ovrd=off  block_type=delay
      settings: xl_area=[17 33 0 33 0 0 0]  block_version=VER_STRING_GOES_HERE
  curr5 : xbsIndex_r4/Delay  rst=off  infoeditControl=Selection of Reset will increase slice count due to use of real FFs and instead of SRLs  en=off  latency=31  reg_retiming=on  dbl_ovrd=off  block_type=delay
      settings: xl_area=[17 33 0 33 0 0 0]  block_version=VER_STRING_GOES_HERE
  curr6 : xbsIndex_r4/Delay  rst=off  infoeditControl=Selection of Reset will increase slice count due to use of real FFs and instead of SRLs  en=off  latency=10  reg_retiming=on  dbl_ovrd=off  block_type=delay
      settings: xl_area=[17 33 0 33 0 0 0]  block_version=VER_STRING_GOES_HERE
  curr7 : xbsIndex_r4/Delay  rst=off  infoeditControl=Selection of Reset will increase slice count due to use of real FFs and instead of SRLs  en=off  latency=15  reg_retiming=on  dbl_ovrd=off  block_type=delay
      settings: xl_area=[17 33 0 33 0 0 0]  block_version=VER_STRING_GOES_HERE
  curr8 : xbsIndex_r4/Delay  rst=off  infoeditControl=Selection of Reset will increase slice count due to use of real FFs and instead of SRLs  en=off  latency=9  reg_retiming=on  dbl_ovrd=off  block_type=delay
      settings: xl_area=[17 33 0 33 0 0 0]  block_version=VER_STRING_GOES_HERE
  Re_0 : Outport
  wires:
  curr6/1 -> curr12/1
  Convert7/1 -> Scope3/4
  Convert6/1 -> Scope3/3
  Convert5/1 -> Scope1/4
  curr1/1 -> Register1/2
  Constant3/1 -> Register6/1
  Subsystem3/2(Out1) -> Scope1/5, curr5/1, Scope2/1, curr2/1, Isin/1, Relational2/1
  Relational2/1 -> Register6/2
  Constant4/1 -> Relational2/2
  Convert3/1 -> Scope2/5
  curr12/1 -> Single Port RAM/3, Scope3/2
  curr11/1 -> Single Port RAM/1, Scope3/1
  Register2/1 -> Scope1/3, Scope2/4, Mux/1
  Convert4/1 -> Scope2/6
  curr8/1 -> Convert3/1, Mux/2
  Register1/1 -> curr7/1
  Register6/1 -> Isin/6
  Subsystem3/1(Out2) -> Relational1/1, Scope1/1, Relational/1
  Relational/1 -> curr19/1, Scope1/2
  Constant6/1 -> Relational/2
  Mux/1 -> Register12/1
  Isin/1 -> Register10/1
  Constant15/1 -> Mux/3
  Constant11/1 -> Subsystem3/1(In1)
  AddSub/1 -> Register1/1, Single Port RAM/2, Convert6/1
  curr7/1 -> Isin/2, Convert2/1, Isin/5
  Re/1 -> Convert5/1, Register17/1
  curr19/1 -> Register11/1
  curr2/1 -> Scope2/3, Isin/4
  Constant2/1 -> Register9/1
  Convert1/1 -> curr1/1
  rst/1 -> Convert1/1
  Relational1/1 -> curr4/1
  Constant1/1 -> Relational1/2
  curr4/1 -> curr6/1
  curr5/1 -> curr11/1
  Single Port RAM/1 -> Re_0/1, Convert7/1
  Register11/1 -> Register2/1
  Register10/1 -> curr8/1
  Register9/1 -> Isin/3
  Register12/1 -> Convert4/1, AddSub/1
  Register13/1 -> Convert8/1, AddSub/2
  Register17/1 -> Register13/1
  start/1 -> Subsystem3/2(start)
  Convert2/1 -> Scope2/2
  Convert8/1 -> Scope2/7

== system mapp_4_fir_4_str/MUX0/add_21 ==
  note: Isin
  Re : Inport
  rst : Inport  Port=2
  start : Inport  Port=3
  AddSub : xbsIndex_r4/AddSub  mode=Addition  use_carryin=off  use_carryout=off  en=off  latency=11  precision=Full  arith_type=Unsigned  n_bits=16  bin_pt=14  quantization=Truncate  overflow=Wrap  use_behavioral_HDL=off  hw_selection=Fabric  pipelined=off  dbl_ovrd=off  block_type=addsub
  Constant1 : xbsIndex_r4/Constant  const=2  gui_display_data_type=Fixed-point  arith_type=Unsigned  n_bits=2  bin_pt=0  preci_type=Single  exp_width=8  frac_width=24  explicit_period=on  period=1  equ=P=C  opselect=C  inp2=PCIN>>17  opr=+  inp1=P  carry=CIN  dbl_ovrd=off  block_type=constant
      settings: block_version=VER_STRING_GOES_HERE
  Constant11 : xbsIndex_r4/Constant  const=382  gui_display_data_type=Fixed-point  arith_type=Unsigned  n_bits=12  bin_pt=0  preci_type=Single  exp_width=8  frac_width=24  explicit_period=off  period=1  equ=P=C  opselect=C  inp2=PCIN>>17  opr=+  inp1=P  carry=CIN  dbl_ovrd=off  block_type=constant
      settings: block_version=VER_STRING_GOES_HERE
  Constant15 : xbsIndex_r4/Constant  const=0  gui_display_data_type=Floating-point  arith_type=Floating-point  n_bits=48  bin_pt=0  preci_type=Single  exp_width=8  frac_width=24  explicit_period=on  period=1  equ=P=C  opselect=C  inp2=PCIN>>17  opr=+  inp1=P  carry=CIN  dbl_ovrd=off  block_type=constant
      settings: block_version=VER_STRING_GOES_HERE
  Constant2 : xbsIndex_r4/Constant  const=0  gui_display_data_type=Fixed-point  arith_type=Boolean  n_bits=16  bin_pt=14  preci_type=Single  exp_width=8  frac_width=24  explicit_period=on  period=1  equ=P=C  opselect=C  inp2=PCIN>>17  opr=+  inp1=P  carry=CIN  dbl_ovrd=off  block_type=constant
      settings: block_version=VER_STRING_GOES_HERE
  Constant3 : xbsIndex_r4/Constant  const=1  gui_display_data_type=Boolean  arith_type=Boolean  n_bits=5  bin_pt=0  preci_type=Single  exp_width=8  frac_width=24  explicit_period=off  period=1  equ=P=C  opselect=C  inp2=PCIN>>17  opr=+  inp1=P  carry=CIN  dbl_ovrd=off  block_type=constant
      settings: block_version=VER_STRING_GOES_HERE
  Constant4 : xbsIndex_r4/Constant  const=1  gui_display_data_type=Fixed-point  arith_type=Unsigned  n_bits=1  bin_pt=0  preci_type=Single  exp_width=8  frac_width=24  explicit_period=off  period=1  equ=P=C  opselect=C  inp2=PCIN>>17  opr=+  inp1=P  carry=CIN  dbl_ovrd=off  block_type=constant
      settings: block_version=VER_STRING_GOES_HERE
  Constant6 : xbsIndex_r4/Constant  const=3  gui_display_data_type=Fixed-point  arith_type=Unsigned  n_bits=2  bin_pt=0  preci_type=Single  exp_width=8  frac_width=24  explicit_period=on  period=1  equ=P=C  opselect=C  inp2=PCIN>>17  opr=+  inp1=P  carry=CIN  dbl_ovrd=off  block_type=constant
      settings: block_version=VER_STRING_GOES_HERE
  Constant8 : xbsIndex_r4/Constant  const=1  gui_display_data_type=Fixed-point  arith_type=Boolean  n_bits=16  bin_pt=14  preci_type=Single  exp_width=8  frac_width=24  explicit_period=on  period=1  equ=P=C  opselect=C  inp2=PCIN>>17  opr=+  inp1=P  carry=CIN  dbl_ovrd=off  block_type=constant
      settings: block_version=VER_STRING_GOES_HERE
  Convert1 : xbsIndex_r4/Convert  gui_display_data_type=Fixed-point  arith_type=Boolean  n_bits=48  bin_pt=48  float_type=Single  exp_bits=8  fraction_bits=24  quantization=Truncate  overflow=Saturate  en=off  latency=0  pipeline=off  dbl_ovrd=off  block_type=convert
      settings: xl_area=[0 0 0 0 0 0 0]  block_version=8.2-EVAL
  Convert{2..8} (7 alike) : xbsIndex_r4/Convert  gui_display_data_type=Floating-point  arith_type=Floating-point  n_bits=16  bin_pt=14  float_type=Single  exp_bits=8  fraction_bits=24  quantization=Truncate  overflow=Wrap  en=off  latency=0  pipeline=off  dbl_ovrd=off  block_type=convert
  Isin : xbsIndex_r4/Dual Port RAM  depth=num_harm_32  initVector=zeros  distributed_mem=Block RAM  init_a=0  init_b=0  rst_a=off  rst_b=off  en_a=off  en_b=off  latency=1  write_mode_A=Read Before Write  write_mode_B=Read Before Write  optimize=Speed  dbl_ovrd=off  block_type=dpram
      settings: xl_area=[96 48 48 144 0 0 0]  block_version=VER_STRING_GOES_HERE
  Mux : xbsIndex_r4/Mux  inputs=2  en=off  latency=0  precision=Full  arith_type=Unsigned  n_bits=16  bin_pt=14  quantization=Truncate  overflow=Wrap  dbl_ovrd=off  block_type=mux
  Register1 : xbsIndex_r4/Register  init=0  rst=on  en=off  dbl_ovrd=off  block_type=register
      settings: xl_area=[18 36 0 0 0 0 0]  block_version=VER_STRING_GOES_HERE
  Register{2,9..13,17} (7 alike) : xbsIndex_r4/Register  init=0  rst=off  en=off  dbl_ovrd=off  block_type=register
  Register6 : xbsIndex_r4/Register  init=0  rst=off  en=on  dbl_ovrd=off  block_type=register
  Relational : xbsIndex_r4/Relational  mode=a=b  op_type=Bool  en=off  latency=0  dbl_ovrd=off  block_type=relational
  Relational1 : xbsIndex_r4/Relational  mode=a=b  op_type=Bool  en=off  latency=0  dbl_ovrd=off  block_type=relational
  Relational2 : xbsIndex_r4/Relational  mode=a=b  op_type=Bool  en=off  latency=1  dbl_ovrd=off  block_type=relational
      settings: xl_area=[4 1 0 7 0 0 0]  block_version=VER_STRING_GOES_HERE
  Scope1 : Scope  NumInputPorts=6
  Scope2 : Scope  NumInputPorts=7
  Scope3 : Scope  NumInputPorts=6
  Single Port RAM : xbsIndex_r4/Single Port RAM  depth=num_harm_32  initVector=zeros  distributed_mem=Block RAM  write_mode=Read After Write  rst=off  init_reg=0  en=off  latency=1  optimize=Area  dbl_ovrd=off  block_type=spram
  Subsystem3 : Subsystem
  curr1 : xbsIndex_r4/Delay  rst=off  infoeditControl=Selection of Reset will increase slice count due to use of real FFs and instead of SRLs  en=off  latency=5  reg_retiming=on  dbl_ovrd=off  block_type=delay
      settings: xl_area=[17 33 0 33 0 0 0]  block_version=VER_STRING_GOES_HERE
  curr11 : xbsIndex_r4/Delay  rst=off  infoeditControl=Selection of Reset will increase slice count due to use of real FFs and instead of SRLs  en=off  latency=1  reg_retiming=on  dbl_ovrd=off  block_type=delay
      settings: xl_area=[17 33 0 33 0 0 0]  block_version=VER_STRING_GOES_HERE
  curr12 : xbsIndex_r4/Delay  rst=off  infoeditControl=Selection of Reset will increase slice count due to use of real FFs and instead of SRLs  en=off  latency=1  reg_retiming=on  dbl_ovrd=off  block_type=delay
      settings: xl_area=[17 33 0 33 0 0 0]  block_version=VER_STRING_GOES_HERE
  curr19 : xbsIndex_r4/Delay  rst=off  infoeditControl=Selection of Reset will increase slice count due to use of real FFs and instead of SRLs  en=off  latency=18  reg_retiming=on  dbl_ovrd=off  block_type=delay
      settings: xl_area=[17 33 0 33 0 0 0]  block_version=VER_STRING_GOES_HERE
  curr2 : xbsIndex_r4/Delay  rst=off  infoeditControl=Selection of Reset will increase slice count due to use of real FFs and instead of SRLs  en=off  latency=39  reg_retiming=on  dbl_ovrd=off  block_type=delay
      settings: xl_area=[17 33 0 33 0 0 0]  block_version=VER_STRING_GOES_HERE
  curr4 : xbsIndex_r4/Delay  rst=off  infoeditControl=Selection of Reset will increase slice count due to use of real FFs and instead of SRLs  en=off  latency=21  reg_retiming=on  dbl_ovrd=off  block_type=delay
      settings: xl_area=[17 33 0 33 0 0 0]  block_version=VER_STRING_GOES_HERE
  curr5 : xbsIndex_r4/Delay  rst=off  infoeditControl=Selection of Reset will increase slice count due to use of real FFs and instead of SRLs  en=off  latency=31  reg_retiming=on  dbl_ovrd=off  block_type=delay
      settings: xl_area=[17 33 0 33 0 0 0]  block_version=VER_STRING_GOES_HERE
  curr6 : xbsIndex_r4/Delay  rst=off  infoeditControl=Selection of Reset will increase slice count due to use of real FFs and instead of SRLs  en=off  latency=10  reg_retiming=on  dbl_ovrd=off  block_type=delay
      settings: xl_area=[17 33 0 33 0 0 0]  block_version=VER_STRING_GOES_HERE
  curr7 : xbsIndex_r4/Delay  rst=off  infoeditControl=Selection of Reset will increase slice count due to use of real FFs and instead of SRLs  en=off  latency=15  reg_retiming=on  dbl_ovrd=off  block_type=delay
      settings: xl_area=[17 33 0 33 0 0 0]  block_version=VER_STRING_GOES_HERE
  curr8 : xbsIndex_r4/Delay  rst=off  infoeditControl=Selection of Reset will increase slice count due to use of real FFs and instead of SRLs  en=off  latency=9  reg_retiming=on  dbl_ovrd=off  block_type=delay
      settings: xl_area=[17 33 0 33 0 0 0]  block_version=VER_STRING_GOES_HERE
  Re_0 : Outport
  wires:
  Convert8/1 -> Scope2/7
  Convert2/1 -> Scope2/2
  start/1 -> Subsystem3/2(start)
  Register17/1 -> Register13/1
  Register13/1 -> AddSub/2, Convert8/1
  Register12/1 -> AddSub/1, Convert4/1
  Register9/1 -> Isin/3
  Register10/1 -> curr8/1
  Register11/1 -> Register2/1
  Single Port RAM/1 -> Convert7/1, Re_0/1
  curr5/1 -> curr11/1
  curr4/1 -> curr6/1
  Constant1/1 -> Relational1/2
  Relational1/1 -> curr4/1
  rst/1 -> Convert1/1
  Convert1/1 -> curr1/1
  Constant2/1 -> Register9/1
  curr2/1 -> Isin/4, Scope2/3
  curr19/1 -> Register11/1
  Re/1 -> Register17/1, Convert5/1
  curr7/1 -> Isin/5, Convert2/1, Isin/2
  AddSub/1 -> Convert6/1, Single Port RAM/2, Register1/1
  Constant11/1 -> Subsystem3/1(In1)
  Constant15/1 -> Mux/3
  Isin/1 -> Register10/1
  Mux/1 -> Register12/1
  Constant6/1 -> Relational/2
  Relational/1 -> Scope1/2, curr19/1
  Subsystem3/1(Out2) -> Relational/1, Scope1/1, Relational1/1
  Register6/1 -> Isin/6
  Register1/1 -> curr7/1
  curr8/1 -> Mux/2, Convert3/1
  Convert4/1 -> Scope2/6
  Register2/1 -> Mux/1, Scope2/4, Scope1/3
  curr11/1 -> Scope3/1, Single Port RAM/1
  curr12/1 -> Scope3/2, Single Port RAM/3
  Convert3/1 -> Scope2/5
  Constant4/1 -> Relational2/2
  Relational2/1 -> Register6/2
  Subsystem3/2(Out1) -> Relational2/1, Isin/1, curr2/1, Scope2/1, curr5/1, Scope1/5
  Constant3/1 -> Register6/1
  curr1/1 -> Register1/2
  Convert5/1 -> Scope1/4
  Convert6/1 -> Scope3/3
  Convert7/1 -> Scope3/4
  curr6/1 -> curr12/1

== system mapp_4_fir_4_str/MUX0/ci_re_0 ==
  addr : Inport
  m_data : Inport  Port=2
  m_addr : Inport  Port=3
  m_en : Inport  Port=4
  Convert2 : xbsIndex_r4/Convert  gui_display_data_type=Floating-point  arith_type=Floating-point  n_bits=16  bin_pt=14  float_type=Single  exp_bits=8  fraction_bits=24  quantization=Truncate  overflow=Wrap  en=off  latency=6  pipeline=off  dbl_ovrd=off  block_type=convert
  Delay{1..5} (5 alike) : xbsIndex_r4/Delay  rst=off  infoeditControl=Selection of Reset will increase slice count due to use of real FFs and instead of SRLs  en=off  latency=1  reg_retiming=off  dbl_ovrd=off  block_type=delay
  Mux1 : xbsIndex_r4/Mux  inputs=2  en=off  latency=0  precision=Full  arith_type=Unsigned  n_bits=16  bin_pt=14  quantization=Truncate  overflow=Wrap  dbl_ovrd=off  block_type=mux
  Reinterpret9 : xbsIndex_r4/Reinterpret  force_arith_type=on  arith_type=Floating-point  force_bin_pt=on  bin_pt=24  block_type=reinterpret
  Relational14 : xbsIndex_r4/Relational  mode=a=b  op_type=Bool  en=off  latency=0  dbl_ovrd=off  block_type=relational
  Single Port RAM2 : xbsIndex_r4/Single Port RAM  depth=1024  initVector=Res1  distributed_mem=Block RAM  write_mode=Read After Write  rst=off  init_reg=0  en=off  latency=1  optimize=Area  dbl_ovrd=off  block_type=spram
  re_0 : xbsIndex_r4/Constant  const=CMD_ci_Re_0  gui_display_data_type=Fixed-point  arith_type=Unsigned  n_bits=8  bin_pt=0  preci_type=Single  exp_width=8  frac_width=24  explicit_period=on  period=1  equ=P=C  opselect=C  inp2=PCIN>>17  opr=+  inp1=P  carry=CIN  dbl_ovrd=off  block_type=constant
      settings: block_version=VER_STRING_GOES_HERE
  Out : Outport
  wires:
  Delay5/1 -> Single Port RAM2/3, Mux1/1
  Delay1/1 -> Single Port RAM2/2
  Delay4/1 -> Out/1
  Single Port RAM2/1 -> Delay2/1
  Convert2/1 -> Delay4/1
  Delay2/1 -> Reinterpret9/1
  Reinterpret9/1 -> Delay3/1
  Delay3/1 -> Convert2/1
  Mux1/1 -> Single Port RAM2/1
  re_0/1 -> Relational14/2
  Relational14/1 -> Delay5/1
  addr/1 -> Mux1/2
  m_en/1 -> Relational14/1
  m_addr/1 -> Mux1/3
  m_data/1 -> Delay1/1
